simulink model "ReducedObserver"  (R2017a)
settings: Solver=VariableStepAuto  StartTime=0.0  StopTime=10.0  RelTol=1e-3
undefined symbols (not defined in the file): A, Aq, B, Bq, c, C, D, F, K1, Kq, L1, L2, m, n, x0, x0hat_reduced
settings Model: Creator=AMAN  LastModifiedBy=Amit

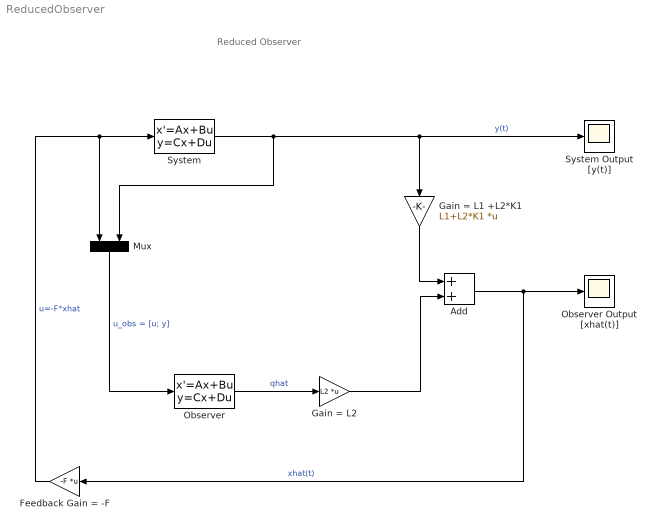
== system ReducedObserver ==
  note: Reduced Observer
  Add : Sum
  Feedback Gain = -F : Gain  Gain=-F  Multiplication=Matrix(K*u)
  Gain = L1 +L2*K1 : Gain  Gain=L1+L2*K1  Multiplication=Matrix(K*u)
  Gain = L2 : Gain  Gain=L2  Multiplication=Matrix(K*u)
  Mux : Mux  Inputs=2
  Observer : StateSpace  A=Aq  B=[Bq Kq]  C=eye(n-c)  D=zeros(n-c,m+c)  X0=x0hat_reduced
  Observer Output [xhat(t)] : Scope
  System : StateSpace  A=A  B=B  C=C  D=D  X0=x0
  System Output [y(t)] : Scope
  wires:
  System/1 -> Mux/2, System Output [y(t)]/1, Gain = L1 +L2*K1/1  "y(t)"
  Feedback Gain = -F/1 -> Mux/1, System/1  "u=-F*xhat"
  Mux/1 -> Observer/1  "u_obs = [u; y]"
  Observer/1 -> Gain = L2/1  "qhat"
  Gain = L2/1 -> Add/2
  Gain = L1 +L2*K1/1 -> Add/1
  Add/1 -> Observer Output [xhat(t)]/1, Feedback Gain = -F/1  "xhat(t)"
